simulink model "subsystem"  (R2018a)
settings: Solver=VariableStepAuto  StartTime=0.0  StopTime=10.0  RelTol=1e-3
libraries: dsparch4 x2, commrandsrc3 x2
settings Model: Creator=hp  LastModifiedBy=hp

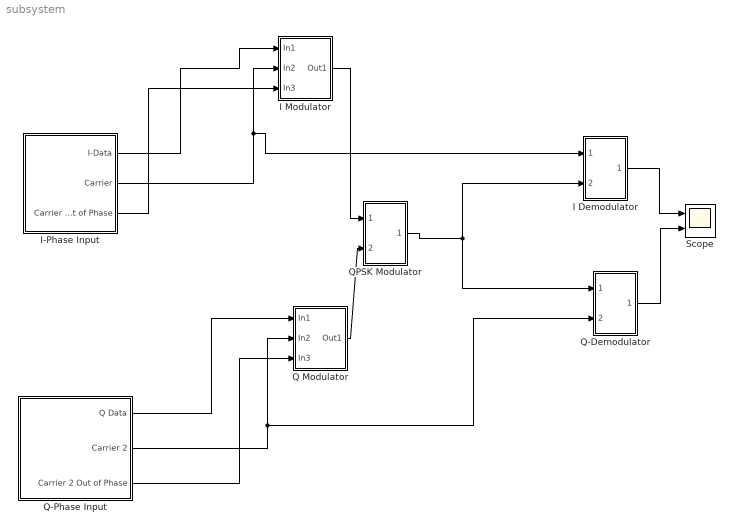
== system subsystem ==
  "I Demodulator " : Subsystem
  I Modulator : Subsystem
  "I-Phase Input " : Subsystem
  Q Modulator : Subsystem
  Q-Demodulator : Subsystem
  Q-Phase Input : Subsystem
  QPSK Modulator : Subsystem
  Scope : Scope  NumInputPorts=2
  wires:
  "I-Phase Input "/2(Carrier) -> "I Demodulator "/1(In1), I Modulator/2(In2)
  "I-Phase Input "/1(I-Data) -> I Modulator/1(In1)
  Q-Phase Input/1(Q Data) -> Q Modulator/1(In1)
  Q-Phase Input/2("Carrier 2 ") -> Q-Demodulator/2(In2), Q Modulator/2(In2)
  I Modulator/1(Out1) -> QPSK Modulator/1(In1)
  "I-Phase Input "/3("Carrier Out of Phase ") -> I Modulator/3(In3)
  Q Modulator/1(Out1) -> QPSK Modulator/2(In2)
  Q-Phase Input/3(Carrier 2 Out of Phase) -> Q Modulator/3(In3)
  QPSK Modulator/1(Out1) -> Q-Demodulator/1(In1), "I Demodulator "/2(In2)
  "I Demodulator "/1(Out1) -> Scope/1
  Q-Demodulator/1(Out1) -> Scope/2

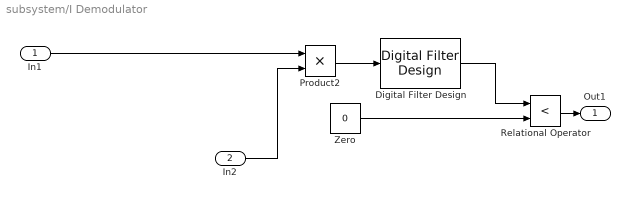
== system subsystem/I Demodulator  ==
  In1 : Inport
  In2 : Inport  Port=2
  Digital Filter Design : dsparch4/Digital Filter Design  mwdsp_browser_bugfix_var=off
  Product2 : Product
  Relational Operator : RelationalOperator  Operator=<  OutDataTypeStr=boolean  RndMeth=Simplest
  Zero : Constant  Value=0
  Out1 : Outport
  wires:
  Digital Filter Design/1 -> Relational Operator/1
  In2/1 -> Product2/2
  Product2/1 -> Digital Filter Design/1
  Zero/1 -> Relational Operator/2
  In1/1 -> Product2/1
  Relational Operator/1 -> Out1/1

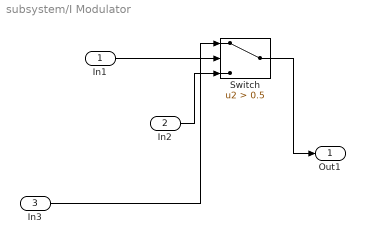
== system subsystem/I Modulator ==
  In1 : Inport
  In2 : Inport  Port=2
  In3 : Inport  Port=3
  Switch : Switch  Criteria=u2 > Threshold  Threshold=0.5
  Out1 : Outport
  wires:
  In3/1 -> Switch/1
  In2/1 -> Switch/3
  Switch/1 -> Out1/1
  In1/1 -> Switch/2

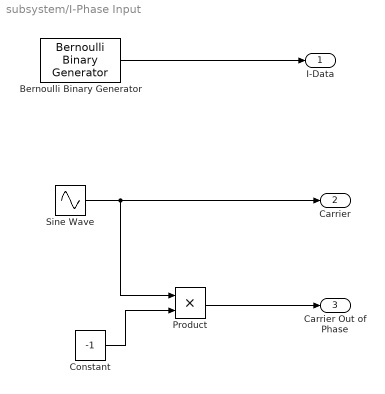
== system subsystem/I-Phase Input  ==
  Bernoulli Binary Generator : commrandsrc3/Bernoulli Binary Generator  ProbabilityOfZero=0.5  SeedSource=Parameter  Seed=60  SampleTime=1  SamplesPerFrame=1  OutputDataType=double  SimulateUsing=Interpreted execution
  Constant : Constant  Value=-1
  Product : Product
  Sine Wave : Sin  Frequency=2*pi*10  SampleTime=0.001
  I-Data : Outport
  Carrier : Outport  Port=2
  "Carrier Out of Phase " : Outport  Port=3
  wires:
  Bernoulli Binary Generator/1 -> I-Data/1
  Sine Wave/1 -> Product/1, Carrier/1
  Constant/1 -> Product/2
  Product/1 -> "Carrier Out of Phase "/1

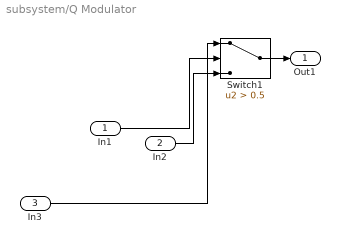
== system subsystem/Q Modulator ==
  In1 : Inport
  In2 : Inport  Port=2
  In3 : Inport  Port=3
  Switch1 : Switch  Criteria=u2 > Threshold  Threshold=0.5
  Out1 : Outport
  wires:
  In1/1 -> Switch1/2
  In3/1 -> Switch1/1
  Switch1/1 -> Out1/1
  In2/1 -> Switch1/3

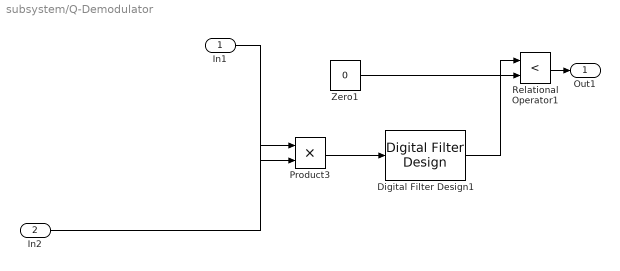
== system subsystem/Q-Demodulator ==
  In1 : Inport
  In2 : Inport  Port=2
  Digital Filter Design1 : dsparch4/Digital Filter Design  mwdsp_browser_bugfix_var=off
  Product3 : Product
  Relational Operator1 : RelationalOperator  Operator=<  OutDataTypeStr=boolean  RndMeth=Simplest
  Zero1 : Constant  Value=0
  Out1 : Outport
  wires:
  Zero1/1 -> Relational Operator1/2
  Digital Filter Design1/1 -> Relational Operator1/1
  Product3/1 -> Digital Filter Design1/1
  In2/1 -> Product3/1
  Relational Operator1/1 -> Out1/1
  In1/1 -> Product3/2

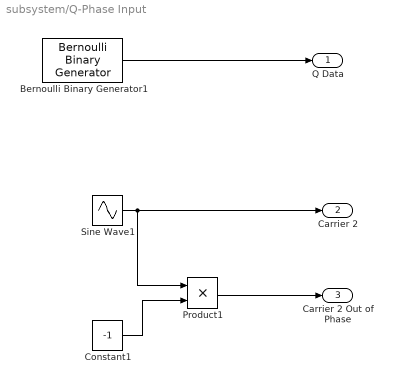
== system subsystem/Q-Phase Input ==
  Bernoulli Binary Generator1 : commrandsrc3/Bernoulli Binary Generator  ProbabilityOfZero=0.5  SeedSource=Parameter  Seed=60  SampleTime=1  SamplesPerFrame=1  OutputDataType=double  SimulateUsing=Interpreted execution
  Constant1 : Constant  Value=-1
  Product1 : Product
  Sine Wave1 : Sin  Frequency=2*pi*2  Phase=pi/2  SampleTime=0.001
  Q Data : Outport
  "Carrier 2 " : Outport  Port=2
  Carrier 2 Out of Phase : Outport  Port=3
  wires:
  Constant1/1 -> Product1/2
  Sine Wave1/1 -> Product1/1, "Carrier 2 "/1
  Bernoulli Binary Generator1/1 -> Q Data/1
  Product1/1 -> Carrier 2 Out of Phase/1

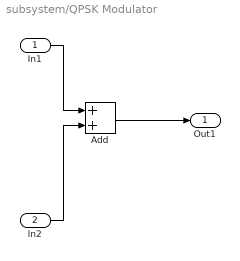
== system subsystem/QPSK Modulator ==
  In1 : Inport
  In2 : Inport  Port=2
  Add : Sum
  Out1 : Outport
  wires:
  In2/1 -> Add/2
  In1/1 -> Add/1
  Add/1 -> Out1/1
